simulink model "section_4_3"  (R2021b)
settings: Solver=VariableStepAuto  StartTime=0.0  StopTime=1000  RelTol=1e-3
values from neighbouring files (symbols this model uses):
  Pz_new_den = cell2mat(Pz_new.Denominator)    [lab3.m]
  Pz_new_num = cell2mat(Pz_new.Numerator)    [lab3.m]
  T = 0.1    [lab3.m]
settings Model: Creator=varunsampat  LastModifiedBy=varunsampat

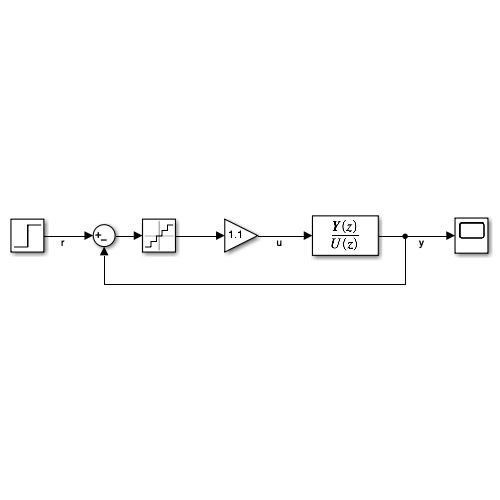
[thumbnail: Simulink's stored preview of the top-level diagram]
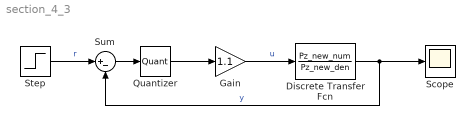
== system section_4_3 ==
  Discrete Transfer Fcn : DiscreteTransferFcn  Numerator=Pz_new_num  Denominator=Pz_new_den  SampleTime=T
  Gain : Gain  Gain=1.1
  Quantizer : Quantizer  QuantizationInterval=0.2
  Scope : Scope
  Step : Step  SampleTime=0
  Sum : Sum  Inputs=|+-
  wires:
  Gain/1 -> Discrete Transfer Fcn/1  "u"
  Discrete Transfer Fcn/1 -> Scope/1, Sum/2  "y"
  Step/1 -> Sum/1  "r"
  Sum/1 -> Quantizer/1
  Quantizer/1 -> Gain/1
